simulink model "LinearTopObserverDisc"  (R2019a)
settings: Solver=FixedStepAuto  StartTime=0.0  StopTime=0.5  FixedStep=h  RelTol=1e-3
values from neighbouring files (symbols this model uses):
  Parameters = [0  0; 0  0]    [matlab.mat]
undefined symbols (not defined in the file or in its folder): DiscIntNeverNeededParam
settings Model: Creator=coeng  LastModifiedBy=coeng
settings DebuggingCC: ArithmeticOperatorsInVariantConditions=warning
settings CodeAppCC: StateflowObjectComments=on

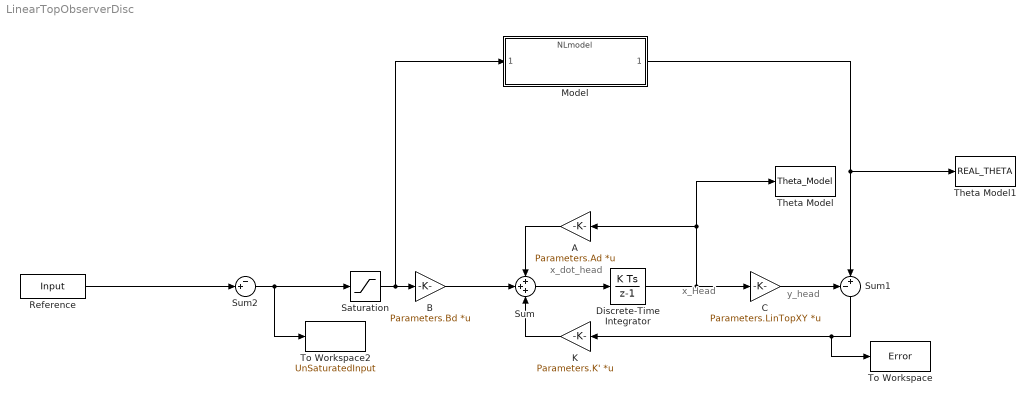
== system LinearTopObserverDisc ==
  note: y_head
  note: x_dot_head
  note: x_Head
  A : Gain  Gain=Parameters.Ad  Multiplication=Matrix(K*u)
  B : Gain  Gain=Parameters.Bd  Multiplication=Matrix(K*u)
  C : Gain  Gain=Parameters.LinTopXY  Multiplication=Matrix(K*u)
  Discrete-Time Integrator : DiscreteIntegrator  SampleTime=-1  ICPrevOutput=DiscIntNeverNeededParam  ICPrevScaledInput=DiscIntNeverNeededParam
  K : Gain  Gain=Parameters.K'  Multiplication=Matrix(K*u)
  Model : ModelReference  ModelNameDialog=NLmodel  SimulationMode=Normal  ModelReferenceVersion=1.67
  "Reference " : FromWorkspace  VariableName=Input  SampleTime=0
  Saturation : Saturate  UpperLimit=1  LowerLimit=-1
  Sum : Sum  Inputs=+++
  Sum1 : Sum  Inputs=-+|
  Sum2 : Sum  Inputs=-+|
  Theta Model : ToWorkspace  VariableName=Theta_Model  SaveFormat=Timeseries  SampleTime=-1
  Theta Model1 : ToWorkspace  VariableName=REAL_THETA  SaveFormat=Timeseries  SampleTime=-1
  To Workspace : ToWorkspace  VariableName=Error  SaveFormat=Timeseries  SampleTime=-1
  To Workspace2 : ToWorkspace  VariableName=UnSaturatedInput  SaveFormat=Timeseries  SampleTime=-1
  wires:
  Sum/1 -> Discrete-Time Integrator/1
  Discrete-Time Integrator/1 -> A/1, Theta Model/1, C/1
  Sum2/1 -> To Workspace2/1, Saturation/1
  Saturation/1 -> Model/1, B/1
  Sum1/1 -> K/1, To Workspace/1
  K/1 -> Sum/3
  C/1 -> Sum1/1
  A/1 -> Sum/1
  B/1 -> Sum/2
  "Reference "/1 -> Sum2/2
  Model/1 -> Theta Model1/1, Sum1/2
